simulink model "fossen_control"  (R2023b)
settings: Solver=VariableStepAuto  StartTime=0.0  StopTime=1000  RelTol=1e-3
undefined symbols (not defined in the file): desired_eta_dot, eta_t_0, m, q, random_current, speed_0, x, y
libraries: simulink x1
settings Model: Creator=ambra  LastModifiedBy=ambra

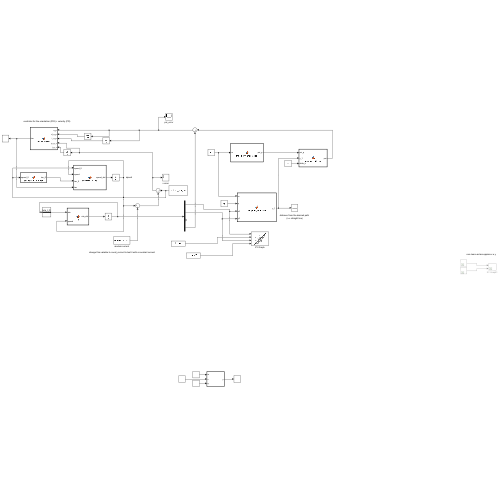
[thumbnail: Simulink's stored preview of the top-level diagram]
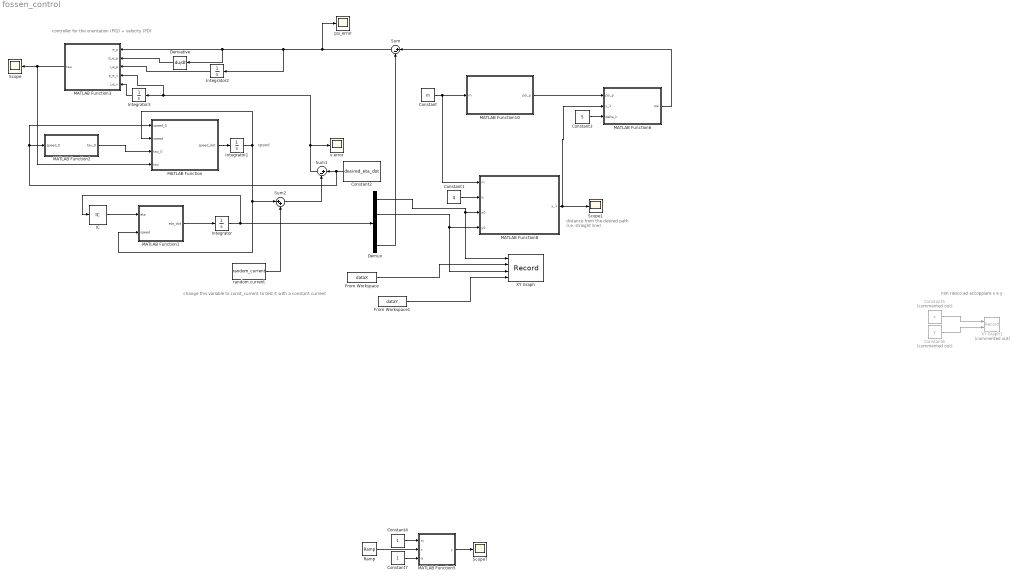
== system fossen_control ==
  note: change this variable to const_current to test it with a constant current
  note: distance from the desired path
      | (i.e. straight line)
  note: non riesco ad accoppiare x e y
  note: controller for the orientation (PID) + velocity (PD)
  note: speed
  Constant : Constant  Value=m
  Constant1 : Constant  Value=q
  Constant2 : Constant  Value=desired_eta_dot
  Constant3 : Constant  Value=5
  Constant4 : Constant
  Constant5 : Constant  Commented=on  Value=x
  Constant6 : Constant  Commented=on  Value=y
  Constant7 : Constant
  Demux : Demux
  Derivative : Derivative
  From Workspace : FromWorkspace  VariableName=dataX  SampleTime=-1
  From Workspace1 : FromWorkspace  VariableName=dataY  SampleTime=-1
  IC : InitialCondition  Value=eta_t_0
  Integrator : Integrator  InitialCondition=eta_t_0
  Integrator1 : Integrator  InitialCondition=speed_0
  Integrator2 : Integrator
  Integrator3 : Integrator
  MATLAB Function : MATLAB Function  TreatAsAtomicUnit=on
  MATLAB Function1 : MATLAB Function  TreatAsAtomicUnit=on
  MATLAB Function10 : MATLAB Function  TreatAsAtomicUnit=on
  MATLAB Function2 : MATLAB Function  TreatAsAtomicUnit=on
  MATLAB Function3 : MATLAB Function  TreatAsAtomicUnit=on
  MATLAB Function5 : MATLAB Function  TreatAsAtomicUnit=on
  MATLAB Function6 : MATLAB Function  TreatAsAtomicUnit=on
  MATLAB Function8 : MATLAB Function  TreatAsAtomicUnit=on
  Ramp : simulink/Sources/Ramp  slope=1  start=0  InitialOutput=0
  Scope : Scope
  Scope1 : Scope
  Scope7 : Scope
  Sum : Sum  Inputs=|+-
  Sum1 : Sum  Inputs=|+-
  Sum2 : Sum  Inputs=|++
  XY Graph : Record  FileSettingsInternal="{\"entries\":[{\"content\":{\"excelSettings\":{\"content\":{},\"type\":\"Streamout.ExcelSettings\"}},\"type\":\"Streamout.FileSettingStorage\",\"uuid\":\"\"}],\"packageUris\":[\"http:\\/\\/schema.mathworks.com\\/mf0\\/streamout_blocks\\/R2020a\"],\"version\":\"1.0\"}"  Layout=[1 1]  SignalsInternal="{\"entries\":[{\"content\":{\"signals\":[{\"content\":{\"blockPath\":[],\"dimensions\":[1,1],\"domain\":\"\",\"lineColor\":\"#77ac30\",\"plots\":[1],\"port\":1,\"sid\":[\"\"],\"signalID\":2168,\"signalName\":\"Demux:1\"},\"type\":\"RecordBlkView.Signal\",\"uuid\":\"\"},{\"content\":{\"blockPath\":[],\"dimensions\":[1],\"domain\":\"\",\"lineColor\":\"#ff13a6\",\"plots\":[1],\"port\":2,\"sid\":[\"\"],\"signalID\":2172,\"signalName\":\"From\\nWorkspace\"},\"type\":\"RecordBlkView.Signal\",\"uuid\":\"\"},{\"content\":{\"blockPath\":[],\"dimensions\":[1,1],\"domain\":\"\",\"lineColor\":\"#4dbeee\",\"plots\":[1],\"port\":3,\"sid\":[\"\"],\"signalID\":2176,\"signalName\":\"Demux:2\"},\"type\":\"RecordBlkView.Signal\",\"uuid\":\"\"},{\"content\":{\"blockPath\":[],\"dimensions\":[1],\"domain\":\"\",\"lineColor\":\"#d95319\",\"plots\":[1],\"port\":4,\"sid\":[\"\"],\"signalID\":2180,\"signalName\":\"From\\nWorkspace1\"},\"type\":\"RecordBlkView.Signal\",\"uuid\":\"\"}]},\"type\":\"RecordBlkView.InputSignals\",\"uuid\":\"\"}],\"packageUris\":[\"http:\\/\\/schema.mathworks.com\\/mf0\\/streamout_blocks\\/R2020a\"],\"version\":\"1.0\"}"  VisualizationBindings="{\"xyplotplugin\":{\"info\":[{\"series\":[{\"bindingParametersList\":[{\"parameter\":\"X-Axis\",\"signalID\":2168,\"signalName\":\"Demux:1\"},{\"parameter\":\"Y-Axis\",\"signalID\":2176,\"signalName\":\"Demux:2\"}],\"seriesID\":49205},{\"bindingParametersList\":[{\"parameter\":\"X-Axis\",\"signalID\":2172,\"signalName\":\"From\\nWorkspace\"},{\"parameter\":\"Y-Axis\",\"signalID\":2180,\"signalName\":\"From\\nWorkspace1\"}],\"seriesID\":697}],\"subplotID\":1}]}}"  CompatibilityTag=XY
  XY Graph1 : Record  Commented=on  FileSettingsInternal="{\"entries\":[{\"content\":{\"excelSettings\":{\"content\":{},\"type\":\"Streamout.ExcelSettings\"}},\"type\":\"Streamout.FileSettingStorage\",\"uuid\":\"\"}],\"packageUris\":[\"http:\\/\\/schema.mathworks.com\\/mf0\\/streamout_blocks\\/R2020a\"],\"version\":\"1.0\"}"  Layout=[1 1]  SignalsInternal="{\"entries\":[{\"content\":{},\"type\":\"RecordBlkView.InputSignals\",\"uuid\":\"\"}],\"packageUris\":[\"http:\\/\\/schema.mathworks.com\\/mf0\\/streamout_blocks\\/R2020a\"],\"version\":\"1.0\"}"  VisualizationBindings="{\"xyplotplugin\":{\"info\":[{\"series\":[],\"subplotID\":1}]}}"  CompatibilityTag=XY
  psi_error : Scope
  random current : Constant  Value=random_current
  v error : Scope
  wires:
  Sum1/1 -> MATLAB Function3/4(p_e_v), Integrator3/1, v error/1
  MATLAB Function1/1(eta_dot) -> Integrator/1
  Integrator1/1 -> Sum2/1, MATLAB Function1/2(speed), MATLAB Function/2(speed)
  MATLAB Function/1(speed_dot) -> Integrator1/1
  Constant2/1 -> Sum1/1, MATLAB Function/1(speed_0), MATLAB Function2/1(speed_0)
  Integrator/1 -> Demux/1, IC/1
  MATLAB Function2/1(tau_0) -> MATLAB Function/3(tau_0)
  Demux/1 -> XY Graph/1, MATLAB Function8/3(x0)
  Demux/2 -> XY Graph/3, MATLAB Function8/4(y0)
  Integrator2/1 -> MATLAB Function3/3(i_e_p)
  Sum/1 -> psi_error/1, Integrator2/1, Derivative/1, MATLAB Function3/1(e_p)
  MATLAB Function8/1(y_1) -> Scope1/1, MATLAB Function6/2(y_1)
  MATLAB Function3/1(tau) -> MATLAB Function/4(tau), Scope/1
  MATLAB Function10/1(psi_p) -> MATLAB Function6/1(psi_p)
  Constant3/1 -> MATLAB Function6/3(delta_h)
  MATLAB Function6/1(psi) -> Sum/1
  Derivative/1 -> MATLAB Function3/2(d_e_p)
  Constant/1 -> MATLAB Function8/1(m), MATLAB Function10/1(m)
  Constant1/1 -> MATLAB Function8/2(q)
  Constant5/1 -> XY Graph1/1
  Constant6/1 -> XY Graph1/2
  MATLAB Function5/1(y) -> Scope7/1
  Constant4/1 -> MATLAB Function5/1(m)
  Ramp/1 -> MATLAB Function5/2(x)
  Constant7/1 -> MATLAB Function5/3(q)
  Integrator3/1 -> MATLAB Function3/5(i_e_v)
  From Workspace/1 -> XY Graph/2
  From Workspace1/1 -> XY Graph/4
  IC/1 -> MATLAB Function1/1(eta)
  Demux/4 -> Sum/2
  random current/1 -> Sum2/2
  Sum2/1 -> Sum1/2

== matlab function fossen_control/MATLAB Function1 ==
  data: eta input; eta_dot output; speed input
function eta_dot = Q(eta, speed) 
% eta = posizione nell'inertial frame, speed = velocità nel body frame

eta_dot = zeros(4,1);
eta_dot(1) = speed(1)*cos(eta(4)) - speed(2)*sin(eta(4));
eta_dot(2) = speed(1)*sin(eta(4)) + speed(2)*cos(eta(4));
eta_dot(3) = speed(3); % z_inertial == z_body --> stesso frame, quindi la w corrisponde alla z_dot
eta_dot(4) = speed(4); % la yaw_dot == r di nuovo perché non ci sono né pitch né roll (stesso discorso della velocità lungo z)

== matlab function fossen_control/MATLAB Function ==
  data: speed_0 input; speed_dot output; speed input; tau_0 input; tau input
function speed_dot = dynamic_model(speed_0, speed, tau_0, tau) % speed_dot = speed_0_dot + delta_speed_dot

    % speed and speed_dot are in the body frame
    speed_dot = zeros(4,1);
    
    % z_B = -0.36;
    m = 30;
    % B = 39200;
    % I_x = 2507;
    % I_y = 1367;
    I_z = 4.14;
    X_du = -25;
    Y_dv = -2.325;
    Z_dw = -19.4311;
    % K_dp = -89;
    % M_dq = -137;
    N_dr = -8.690;
    X_u = -0.2;
    Y_v = -55.117;
    Z_w = 33.6804; % POTREBBE DARE PROBLEMI
    % K_p = -60;
    % M_q = -130;
    N_r = -4.14;
    X_u_u = -19.5;
    Y_v_v = -147.9;
    Z_w_w = -89.4105; % POTREBBE DARE PROBLEMI
    % K_p_p = -304;
    % M_q_q = -658;
    N_r_r = -6.23;
    
    m_u = m - X_du;
    m_v = m - Y_dv;
    m_w = m - Z_dw;
    % m_p = I_x - K_dp;
    % m_q = I_y - M_dq;
    m_r = I_z - N_dr;
    
    m_u_v = m_u - m_v;
    % m_u_w = m_u - m_w;
    % m_v_w = m_v - m_w;
    % m_p_q = m_p - m_q;
    % m_p_r = m_p - m_r;
    % m_q_r = m_q - m_r;
    
    % d_u = - X_u - X_u_u*abs(dx(1));
    % d_v = - Y_v - Y_v_v*abs(dx(2));
    % d_w = - Z_w - Z_w_w*abs(dx(3));
    % d_p = - K_p - K_p_p*abs(dx(4));
    % d_q = - M_q - M_q_q*abs(dx(5));
    % d_r = - N_r - N_r_r*abs(dx(6));
    % d_r = - N_r - N_r_r*abs(dx(3));
    
    % surge speed_dot
    speed_dot(1) = (X_u + 2*abs(speed_0(1))*X_u_u)*(speed(1)-speed_0(1))/m_u + m_v/m_u*(speed_0(4)*(speed(2)-speed_0(2)) + speed_0(2)*(speed(4))-speed_0(4)) + (tau(1)-tau_0(1));
    % sway speed_dot
    tau(2) = 0; tau_0(2) = 0; % sway not actuated
    speed_dot(2) = -m_u/m_v*(speed_0(4)*(speed(1)-speed_0(1)) + speed_0(1)*(speed(4)-speed_0(4))) + (Y_v + Y_v_v*2*abs(speed_0(2)))/m_v*(speed(2)-speed_0(2));
    % heave speed_dot
    alpha = - Z_w/m_w;
    beta = -Z_w_w/m_w;
    gamma = 1/m_w;
    speed_dot(3) = (alpha + beta*2*abs(speed_0(3)))*(speed(3)-speed_0(3)) + gamma*(tau(3)-tau_0(3));
    % yaw speed_dot
    speed_dot(4) = m_u_v/m_r * (speed_0(2)*(speed(1)-speed_0(1)) + speed_0(1)*(speed(2)-speed_0(2))) + (N_r + N_r_r*2*abs(speed_0(4)))/m_r*(speed(4)-speed_0(4)) + (tau(4)-tau_0(4))/m_r;

== matlab function fossen_control/MATLAB Function2 ==
  data: tau_0 output; speed_0 input
function tau_0 = equilibrium_torques(speed_0)
    
    tau_0 = zeros(4,1);

    % z_B = -0.36;
    m = 30;
    W_plus_B = -0.8339; % POTREBBE DARE PROBLEMI
    % I_x = 2507;
    % I_y = 1367;
    I_z = 4.14;
    X_du = -25;
    Y_dv = -2.325;
    Z_dw = -19.4311;
    % K_dp = -89;
    % M_dq = -137;
    N_dr = -8.690;
    X_u = -0.2;
    Y_v = -55.117;
    Z_w = 33.6804; % POTREBBE DARE PROBLEMI
    % K_p = -60;
    % M_q = -130;
    N_r = -4.14;
    X_u_u = -19.5;
    Y_v_v = -147.9;
    Z_w_w = -89.4105; % POTREBBE DARE PROBLEMI
    % K_p_p = -304;
    % M_q_q = -658;
    N_r_r = -6.23;
    
    m_u = m - X_du;
    m_v = m - Y_dv;
    m_w = m - Z_dw;
    % m_p = I_x - K_dp;
    % m_q = I_y - M_dq;
    m_r = I_z - N_dr;
    
    m_u_v = m_u - m_v;
    % m_u_w = m_u - m_w;
    % m_v_w = m_v - m_w;
    % m_p_q = m_p - m_q;
    % m_p_r = m_p - m_r;
    % m_q_r = m_q - m_r;
    
    % d_u = - X_u - X_u_u*abs(dx(1));
    % d_v = - Y_v - Y_v_v*abs(dx(2));
    % d_w = - Z_w - Z_w_w*abs(dx(3));
    % d_p = - K_p - K_p_p*abs(dx(4));
    % d_q = - M_q - M_q_q*abs(dx(5));
    % d_r = - N_r - N_r_r*abs(dx(6));
    % d_r = - N_r - N_r_r*abs(dx(3));

    alpha = - Z_w/m_w;
    beta = - Z_w_w/m_w;
    gamma = 1/m_w;
    delta = (W_plus_B)/m_w;

    tau_0(1) = - m_v*speed_0(2)*speed_0(4) - X_u*speed_0(1) - X_u_u*abs(speed_0(1))*speed_0(1);
    tau_0(2) = 0; % sway not actuated
    tau_0(3) = -(alpha*speed_0(3)+beta*speed_0(3)*abs(speed_0(3))+delta)/gamma;
    tau_0(4) = -(m_u_v*speed_0(1)*speed_0(2) + N_r*speed_0(4) + N_r_r*speed_0(4)*abs(speed_0(4)));

== matlab function fossen_control/MATLAB Function3 ==
  data: tau output; e_p input; d_e_p input; i_e_p input; p_e_v input; i_e_v input
function tau = PIDcontroller(e_p, d_e_p, i_e_p, p_e_v, i_e_v)
K_p = 30;
K_i = 10;
K_d = 2;
u = e_p*K_p + d_e_p*K_d + i_e_p*K_i;
K_p_v = 40;
K_i_v = 20;
tau_v = p_e_v*K_p_v + i_e_v*K_i_v;
tau = tau_v;
tau(4) = tau(4) + u;
tau(2) = 0; % sway not actuated

== matlab function fossen_control/MATLAB Function5 ==
  data: m input; y output; x input; q input
function y = retta(m,x,q)
    y = m*x+q;

== matlab function fossen_control/MATLAB Function6 ==
  data: psi_p input; psi output; y_1 input; delta_h input
function psi = heading_ctrl_law(psi_p, y_1, delta_h)

    psi = psi_p + atan2(-y_1,delta_h);

== matlab function fossen_control/MATLAB Function8 ==
  data: m input; y_1 output; q input; x0 input; y0 input
function y_1 = compute_distance(m, q, x0, y0)
    y_1 = abs(y0-(m*x0+q))/sqrt(1+m*m);

== matlab function fossen_control/MATLAB Function10 ==
  data: m input; psi_p output
function psi_p = trajectory_orientation(m)
    psi_p = atan(m);
    psi_p = pi/2 - psi_p;
